simulink model "pcc_dynamic_model_actuation_dynamics"  (R2021a)
settings: Solver=VariableStepAuto  StartTime=0.0  StopTime=30  MaxStep=0.005  RelTol=1e-3
libraries: simulink x3, simulink_extras x3, pid_lib x1
settings Model: PauseTimes=0  Creator=maximilianstoelzle  LastModifiedBy=mstolzle

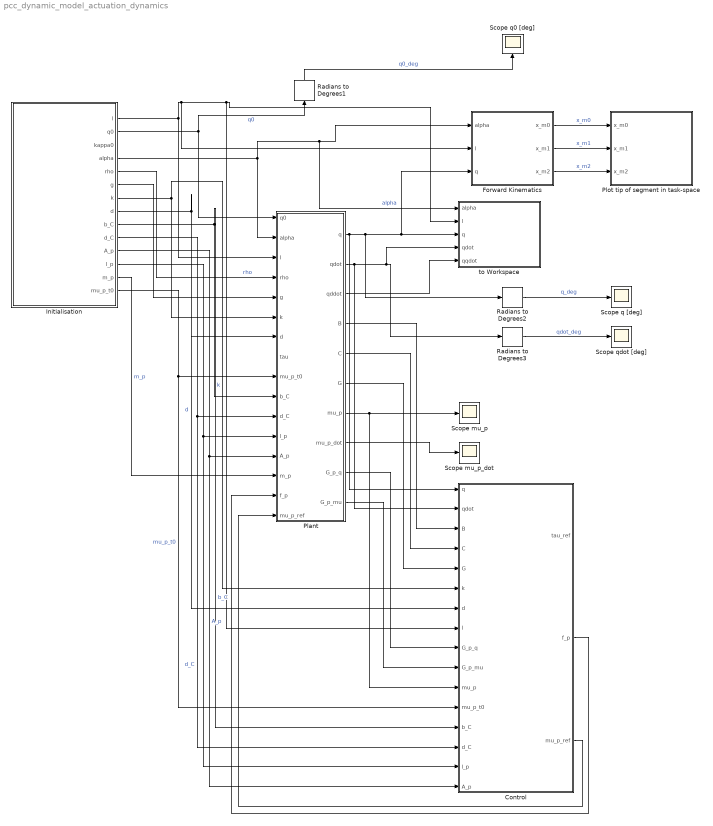
== system pcc_dynamic_model_actuation_dynamics ==
  Control : Subsystem
  Forward Kinematics : MATLAB Function  TreatAsAtomicUnit=on
  Initialisation : Subsystem
  Plant : Subsystem
  Plot tip of segment in task-space : Subsystem
  Radians to Degrees1 : simulink_extras/Transformations/Radians to Degrees
  Radians to Degrees2 : simulink_extras/Transformations/Radians to Degrees
  Radians to Degrees3 : simulink_extras/Transformations/Radians to Degrees
  Scope mu_p : Scope
  Scope mu_p_dot : Scope
  Scope q [deg] : Scope
  Scope q0 [deg] : Scope
  Scope qdot [deg] : Scope
  to Workspace : Subsystem
  wires:
  Initialisation/13(m_p) -> Plant/14(m_p)  "m_p"
  Plant/5(C) -> Control/4(C)
  Control/3(mu_p_ref) -> Plant/16(mu_p_ref)
  Initialisation/14(mu_p_t0) -> Plant/9(mu_p_t0), Control/12(mu_p_t0)  "mu_p_t0"
  Plant/10(G_p_mu) -> Control/10(G_p_mu)
  Initialisation/7(k) -> Plant/6(k), Control/6(k)  "k"
  Plant/8(mu_p_dot) -> Scope mu_p_dot/1
  Plant/9(G_p_q) -> Control/9(G_p_q)
  Control/2(f_p) -> Plant/15(f_p)
  Radians to Degrees1/1 -> Scope q0 [deg]/1  "q0_deg"
  Plant/6(G) -> Control/5(G)
  Plant/4(B) -> Control/3(B)
  Initialisation/6(g) -> Plant/5(g)
  Initialisation/5(rho) -> Plant/4(rho)  "rho"
  Plant/3(qddot) -> to Workspace/5(qqdot)
  Radians to Degrees3/1 -> Scope qdot [deg]/1  "qdot_deg"
  Forward Kinematics/3(x_m2) -> Plot tip of segment in task-space/3(x_m2)  "x_m2"
  Forward Kinematics/2(x_m1) -> Plot tip of segment in task-space/2(x_m1)  "x_m1"
  Forward Kinematics/1(x_m0) -> Plot tip of segment in task-space/1(x_m0)  "x_m0"
  Radians to Degrees2/1 -> Scope q [deg]/1  "q_deg"
  Plant/7(mu_p) -> Scope mu_p/1, Control/11(mu_p)
  Initialisation/12(l_p) -> Plant/12(l_p), Control/15(l_p)
  Initialisation/9(b_C) -> Plant/10(b_C), Control/13(b_C)  "b_C"
  Initialisation/10(d_C) -> Control/14(d_C), Plant/11(d_C)  "d_C"
  Initialisation/11(A_p) -> Control/16(A_p), Plant/13(A_p)  "A_p"
  Initialisation/2(q0) -> Plant/1(q0), Radians to Degrees1/1  "q0"
  Plant/1(q) -> Forward Kinematics/3(q), to Workspace/3(q), Radians to Degrees2/1, Control/1(q)
  Plant/2(qdot) -> to Workspace/4(qdot), Radians to Degrees3/1, Control/2(qdot)
  Initialisation/8(d) -> Control/7(d), Plant/7(d)  "d"
  Initialisation/4(alpha) -> Plant/2(alpha), to Workspace/1(alpha), Forward Kinematics/1(alpha)  "alpha"
  Initialisation/1(l) -> Plant/3(l), to Workspace/2(l), Control/8(l), Forward Kinematics/2(l)

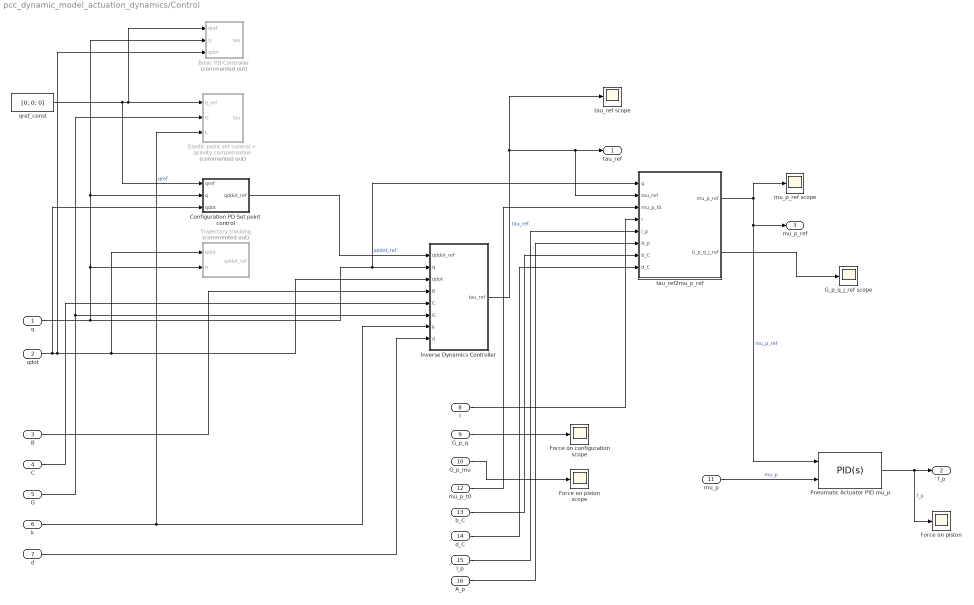
== system pcc_dynamic_model_actuation_dynamics/Control ==
  q : Inport
  qdot : Inport  Port=2
  B : Inport  Port=3
  C : Inport  Port=4
  G : Inport  Port=5
  k : Inport  Port=6
  d : Inport  Port=7
  l : Inport  Port=8
  G_p_q : Inport  Port=9
  G_p_mu : Inport  Port=10
  mu_p : Inport  Port=11
  mu_p_t0 : Inport  Port=12
  b_C : Inport  Port=13
  d_C : Inport  Port=14
  l_p : Inport  Port=15
  A_p : Inport  Port=16
  Basic PD Controller : Subsystem  Commented=on
  Configuration PD Set point control : Subsystem
  Elastic point set control + gravity compensation : MATLAB Function  Commented=on  TreatAsAtomicUnit=on
  Force on configuration scope : Scope
  Force on piston : Scope
  Force on piston scope : Scope
  G_p_q_j_ref scope : Scope
  Inverse Dynamics Controller : MATLAB Function  TreatAsAtomicUnit=on
  Pneumatic Actuator PID mu_p : pid_lib/PID Controller (2DOF)  Controller=PID  Form=Parallel  TimeDomain=Continuous-time  UseExternalTs=off  SampleTime=-1  IntegratorMethod=Forward Euler  FilterMethod=Forward Euler  ControllerParametersSource=internal  P=-3000  I=-500  D=-100  UseFilter=on  N=100  b=1  c=1  TunerSelectOption=Frequency Response Based  InitialConditionSource=internal  InitialConditionForIntegrator=0  InitialConditionForFilter=0  DifferentiatorICPrevScaledInput=0  ExternalReset=none  TrackingMode=off  Kt=1  LimitOutput=off  SatLimitsSource=internal  UpperSaturationLimit=inf  LowerSaturationLimit=-inf  LinearizeAsGain=on  AntiWindupMode=none  Kb=1  POutMin=[]  POutMax=[]  IOutMin=[]  IOutMax=[]  DOutMin=[]  DOutMax=[]  NOutMin=[]  NOutMax=[]  bOutMin=[]  bOutMax=[]  cOutMin=[]  cOutMax=[]  SumOutMin=[]  SumOutMax=[]  SaturationOutMin=[]  SaturationOutMax=[]  PParamMin=[]  PParamMax=[]  IParamMin=[]  IParamMax=[]  DParamMin=[]  DParamMax=[]  NParamMin=[]  NParamMax=[]  bParamMin=[]  bParamMax=[]  cParamMin=[]  cParamMax=[]  KbParamMin=[]  KbParamMax=[]  KtParamMin=[]  KtParamMax=[]  KbOutMin=[]  KbOutMax=[]  KtOutMin=[]  KtOutMax=[]  IntegratorOutMin=[]  IntegratorOutMax=[]  FilterOutMin=[]  FilterOutMax=[]  SumI1OutMin=[]  SumI1OutMax=[]  SumI2OutMin=[]  SumI2OutMax=[]  SumI3OutMin=[]  SumI3OutMax=[]  SumI4OutMin=[]  SumI4OutMax=[]  SumDOutMin=[]  SumDOutMax=[]  Sum1OutMin=[]  Sum1OutMax=[]  Sum2OutMin=[]  Sum2OutMax=[]  Sum3OutMin=[]  Sum3OutMax=[]  DifferentiatorOutMin=[]  DifferentiatorOutMax=[]  FilterDiffOutCoefMin=[]  FilterDiffOutCoefMax=[]  ReciprocalOutMin=[]  ReciprocalOutMax=[]  SumDenOutMin=[]  SumDenOutMax=[]  SumNumOutMin=[]  SumNumOutMax=[]  DivideOutMin=[]  DivideOutMax=[]  UdiffTsProdOutMin=[]  UdiffTsProdOutMax=[]  NTsProdOutMin=[]  NTsProdOutMax=[]  UintegralTsProdOutMin=[]  UintegralTsProdOutMax=[]  UngainTsProdOutMin=[]  UngainTsProdOutMax=[]  IntegratorContinuousStateAttributes=''  IntegratorStateMustResolveToSignalObject=off  IntegratorRTWStateStorageClass=Auto  FilterContinuousStateAttributes=''  FilterStateMustResolveToSignalObject=off  FilterRTWStateStorageClass=Auto  ParallelPVariant=InternalParameters  IdealPVariant=Disabled  IVariant=InternalParameters  DVariant=InternalParameters  bVariant=InternalParameters  cVariant=InternalParameters  IntegratorVariant=Continuous  SatVariant=Disabled  AWVariant=Passthrough  PCopyVariant=Disabled  TRVariant=Disabled  FdbkBlocksVariant=Forward  IdealPFdbkVariant=Disabled  SatFdbkVariant=Disabled  DerivativeFilterVariant=ContFilter  NVariant=InternalParameters  NCopyVariant=Disabled  FilterICVariant=InternalICsFilter  IntegratorICVariant=InternalICs  ExternalResetVariant=Disabled  TRSumVariant=Passthrough  SumFdbkVariant=Disabled  SumVariant=Sum_PID  TsampFilterVariant=InternalTs  TsampNgainVariant=Passthrough  TsampIntegralVariant=Passthrough  ExternalSaturationOutDataTypeStr=Inherit: Same as second input
      settings: SourceProductBaseCode=SL
  Trajectory tracking : Subsystem  Commented=on
  mu_p_ref scope : Scope
  qref_const : Constant  Value=[0; 0; 0]
  tau_ref scope : Scope
  tau_ref2mu_p_ref : MATLAB Function  TreatAsAtomicUnit=on
  tau_ref : Outport
  f_p : Outport  Port=2
  mu_p_ref : Outport  Port=3
  wires:
  q/1 -> Trajectory tracking/2(q), Configuration PD Set point control/2(q), Basic PD Controller/2(q), tau_ref2mu_p_ref/1(q), Inverse Dynamics Controller/2(q)
  qdot/1 -> Trajectory tracking/1(qdot), Inverse Dynamics Controller/3(qdot), Basic PD Controller/3(qdot), Configuration PD Set point control/3(qdot)
  B/1 -> Inverse Dynamics Controller/4(B)
  C/1 -> Inverse Dynamics Controller/5(C)
  G/1 -> Elastic point set control + gravity compensation/2(G), Inverse Dynamics Controller/6(G)
  k/1 -> Elastic point set control + gravity compensation/3(k), Inverse Dynamics Controller/7(k)
  d/1 -> Inverse Dynamics Controller/8(d)
  qref_const/1 -> Basic PD Controller/1(qref), Elastic point set control + gravity compensation/1(q_ref), Configuration PD Set point control/1(qref)  "qref"
  Configuration PD Set point control/1(qddot_ref) -> Inverse Dynamics Controller/1(qddot_ref)  "qddot_ref"
  Inverse Dynamics Controller/1(tau_ref) -> tau_ref2mu_p_ref/2(tau_ref), tau_ref/1, tau_ref scope/1  "tau_ref"
  Pneumatic Actuator PID mu_p/1 -> Force on piston/1, f_p/1  "f_p"
  mu_p/1 -> Pneumatic Actuator PID mu_p/2  "mu_p"
  tau_ref2mu_p_ref/1(mu_p_ref) -> Pneumatic Actuator PID mu_p/1, mu_p_ref/1, mu_p_ref scope/1  "mu_p_ref"
  mu_p_t0/1 -> tau_ref2mu_p_ref/3(mu_p_t0)
  b_C/1 -> tau_ref2mu_p_ref/7(b_C)
  d_C/1 -> tau_ref2mu_p_ref/8(d_C)
  l_p/1 -> tau_ref2mu_p_ref/5(l_p)
  A_p/1 -> tau_ref2mu_p_ref/6(A_p)
  l/1 -> tau_ref2mu_p_ref/4(l)
  tau_ref2mu_p_ref/2(G_p_q_j_ref) -> G_p_q_j_ref scope/1
  G_p_q/1 -> Force on configuration scope/1
  G_p_mu/1 -> Force on piston scope/1

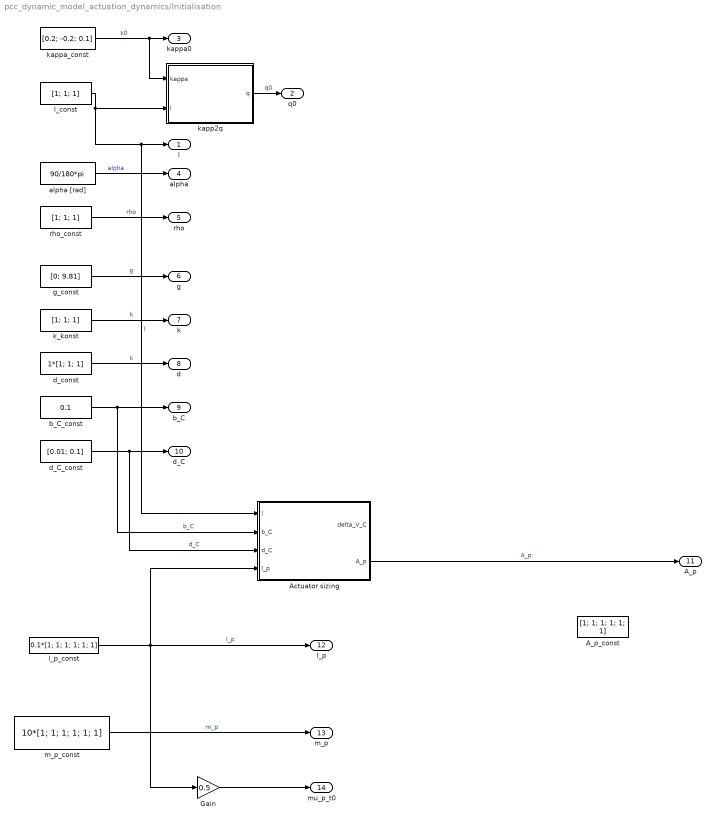
== system pcc_dynamic_model_actuation_dynamics/Initialisation ==
  A_p_const : Constant  Value=[1; 1; 1; 1; 1; 1]
  Actuator sizing : MATLAB Function  TreatAsAtomicUnit=on
  Gain : Gain  Gain=0.5
  alpha [rad] : Constant  Value=90/180*pi
  b_C_const : Constant  Value=0.1
  d_C_const : Constant  Value=[0.01; 0.1]
  d_const : Constant  Value=1*[1; 1; 1]
  g_const : Constant  Value=[0; 9.81]
  k_konst : Constant  Value=[1; 1; 1]
  kapp2q : MATLAB Function  TreatAsAtomicUnit=on
  kappa_const : Constant  Value=[0.2; -0.2; 0.1]
  l_const : Constant  Value=[1; 1; 1]
  l_p_const : Constant  Value=0.1*[1; 1; 1; 1; 1; 1]
  m_p_const : Constant  Value=10*[1; 1; 1; 1; 1; 1]
  rho_const : Constant  Value=[1; 1; 1]
  l : Outport
  q0 : Outport  Port=2
  kappa0 : Outport  Port=3
  alpha : Outport  Port=4
  rho : Outport  Port=5
  g : Outport  Port=6
  k : Outport  Port=7
  d : Outport  Port=8
  b_C : Outport  Port=9
  d_C : Outport  Port=10
  A_p : Outport  Port=11
  l_p : Outport  Port=12
  m_p : Outport  Port=13
  mu_p_t0 : Outport  Port=14
  wires:
  kappa_const/1 -> kapp2q/1(kappa), kappa0/1  "k0"
  l_const/1 -> kapp2q/2(l), Actuator sizing/1(l), l/1  "l"
  alpha [rad]/1 -> alpha/1  "alpha"
  kapp2q/1(q) -> q0/1  "q0"
  rho_const/1 -> rho/1  "rho"
  g_const/1 -> g/1  "g"
  k_konst/1 -> k/1  "k"
  d_const/1 -> d/1  "k"
  d_C_const/1 -> Actuator sizing/3(d_C), d_C/1  "d_C"
  m_p_const/1 -> m_p/1  "m_p"
  b_C_const/1 -> Actuator sizing/2(b_C), b_C/1  "b_C"
  l_p_const/1 -> Gain/1, Actuator sizing/4(l_p), l_p/1  "l_p"
  Actuator sizing/2(A_p) -> A_p/1  "A_p"
  Gain/1 -> mu_p_t0/1

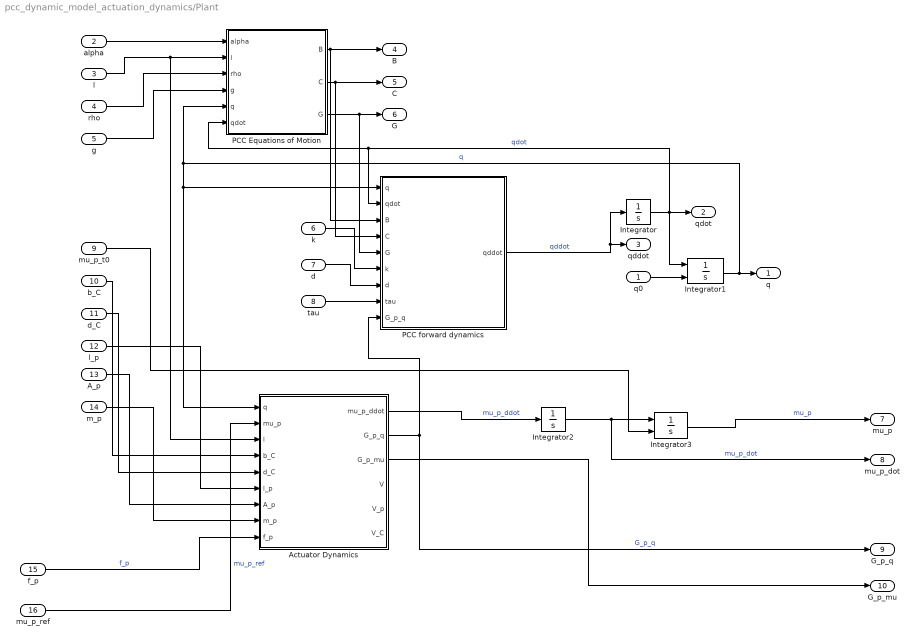
== system pcc_dynamic_model_actuation_dynamics/Plant ==
  q0 : Inport
  alpha : Inport  Port=2
  l : Inport  Port=3
  rho : Inport  Port=4
  g : Inport  Port=5
  k : Inport  Port=6
  d : Inport  Port=7
  tau : Inport  Port=8
  mu_p_t0 : Inport  Port=9
  b_C : Inport  Port=10
  d_C : Inport  Port=11
  l_p : Inport  Port=12
  A_p : Inport  Port=13
  m_p : Inport  Port=14
  f_p : Inport  Port=15
  mu_p_ref : Inport  Port=16
  Actuator Dynamics : MATLAB Function  TreatAsAtomicUnit=on
  Integrator : Integrator  InitialCondition=[0; 0; 0]
  Integrator1 : Integrator  InitialConditionSource=external
  Integrator2 : Integrator  InitialCondition=[0; 0; 0; 0; 0; 0]
  Integrator3 : Integrator  InitialConditionSource=external  LimitOutput=on  UpperSaturationLimit=0.1*[1; 1; 1; 1; 1; 1]  LowerSaturationLimit=[0; 0; 0; 0; 0; 0]
  PCC Equations of Motion : MATLAB Function  TreatAsAtomicUnit=on
  PCC forward dynamics : MATLAB Function  TreatAsAtomicUnit=on
  q : Outport
  qdot : Outport  Port=2
  qddot : Outport  Port=3
  B : Outport  Port=4
  C : Outport  Port=5
  G : Outport  Port=6
  mu_p : Outport  Port=7
  mu_p_dot : Outport  Port=8
  G_p_q : Outport  Port=9
  G_p_mu : Outport  Port=10
  wires:
  g/1 -> PCC Equations of Motion/4(g)
  alpha/1 -> PCC Equations of Motion/1(alpha)
  q0/1 -> Integrator1/2
  k/1 -> PCC forward dynamics/6(k)
  l/1 -> Actuator Dynamics/3(l), PCC Equations of Motion/2(l)
  PCC Equations of Motion/3(G) -> PCC forward dynamics/5(G), G/1
  PCC Equations of Motion/1(B) -> PCC forward dynamics/3(B), B/1
  Integrator1/1 -> PCC Equations of Motion/5(q), Actuator Dynamics/1(q), PCC forward dynamics/1(q), q/1  "q"
  PCC forward dynamics/1(qddot) -> Integrator/1, qddot/1  "qddot"
  rho/1 -> PCC Equations of Motion/3(rho)
  d/1 -> PCC forward dynamics/7(d)
  Integrator/1 -> PCC forward dynamics/2(qdot), PCC Equations of Motion/6(qdot), Integrator1/1, qdot/1  "qdot"
  PCC Equations of Motion/2(C) -> PCC forward dynamics/4(C), C/1
  A_p/1 -> Actuator Dynamics/7(A_p)
  m_p/1 -> Actuator Dynamics/8(m_p)
  Actuator Dynamics/1(mu_p_ddot) -> Integrator2/1  "mu_p_ddot"
  d_C/1 -> Actuator Dynamics/5(d_C)
  Integrator2/1 -> Integrator3/1, mu_p_dot/1  "mu_p_dot"
  b_C/1 -> Actuator Dynamics/4(b_C)
  l_p/1 -> Actuator Dynamics/6(l_p)
  Integrator3/1 -> mu_p/1  "mu_p"
  Actuator Dynamics/2(G_p_q) -> G_p_q/1, PCC forward dynamics/9(G_p_q)  "G_p_q"
  tau/1 -> PCC forward dynamics/8(tau)
  Actuator Dynamics/3(G_p_mu) -> G_p_mu/1
  f_p/1 -> Actuator Dynamics/9(f_p)  "f_p"
  mu_p_t0/1 -> Integrator3/2
  mu_p_ref/1 -> Actuator Dynamics/2(mu_p)  "mu_p_ref"

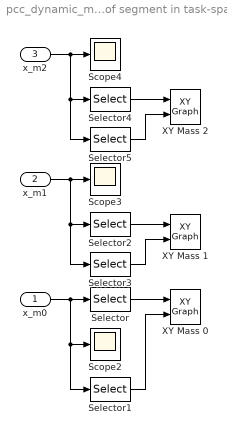
== system pcc_dynamic_model_actuation_dynamics/Plot tip of segment in task-space ==
  x_m0 : Inport
  x_m1 : Inport  Port=2
  x_m2 : Inport  Port=3
  Scope2 : Scope
  Scope3 : Scope
  Scope4 : Scope
  Selector : Selector  InputPortWidth=2  IndexOptions=Index vector (dialog)  Indices=[1]  OutputSizes=1
  Selector1 : Selector  InputPortWidth=2  IndexOptions=Index vector (dialog)  Indices=[2]  OutputSizes=1
  Selector2 : Selector  InputPortWidth=2  IndexOptions=Index vector (dialog)  Indices=[1]  OutputSizes=1
  Selector3 : Selector  InputPortWidth=2  IndexOptions=Index vector (dialog)  Indices=[2]  OutputSizes=1
  Selector4 : Selector  InputPortWidth=2  IndexOptions=Index vector (dialog)  Indices=[1]  OutputSizes=1
  Selector5 : Selector  InputPortWidth=2  IndexOptions=Index vector (dialog)  Indices=[2]  OutputSizes=1
  XY Mass 0 : simulink/Sinks/XY Graph  xmin=-10  xmax=10  ymin=-10  ymax=10  st=-1
  XY Mass 1 : simulink/Sinks/XY Graph  xmin=-10  xmax=10  ymin=-10  ymax=10  st=-1
  XY Mass 2 : simulink/Sinks/XY Graph  xmin=-10  xmax=10  ymin=-10  ymax=10  st=-1
  wires:
  x_m2/1 -> Selector5/1, Selector4/1, Scope4/1
  Selector/1 -> XY Mass 0/1
  x_m1/1 -> Selector3/1, Selector2/1, Scope3/1
  Selector5/1 -> XY Mass 2/2
  Selector3/1 -> XY Mass 1/2
  Selector1/1 -> XY Mass 0/2
  x_m0/1 -> Scope2/1, Selector1/1, Selector/1
  Selector4/1 -> XY Mass 2/1
  Selector2/1 -> XY Mass 1/1

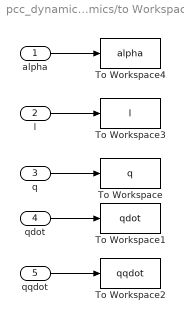
== system pcc_dynamic_model_actuation_dynamics/to Workspace ==
  alpha : Inport
  l : Inport  Port=2
  q : Inport  Port=3
  qdot : Inport  Port=4
  qqdot : Inport  Port=5
  To Workspace : ToWorkspace  VariableName=q  SaveFormat=Timeseries  SampleTime=-1
  To Workspace1 : ToWorkspace  VariableName=qdot  SaveFormat=Timeseries  SampleTime=-1
  To Workspace2 : ToWorkspace  VariableName=qqdot  SaveFormat=Timeseries  SampleTime=-1
  To Workspace3 : ToWorkspace  VariableName=l  SaveFormat=Timeseries  SampleTime=-1
  To Workspace4 : ToWorkspace  VariableName=alpha  SaveFormat=Timeseries  SampleTime=-1
  wires:
  alpha/1 -> To Workspace4/1
  qdot/1 -> To Workspace1/1
  l/1 -> To Workspace3/1
  qqdot/1 -> To Workspace2/1
  q/1 -> To Workspace/1

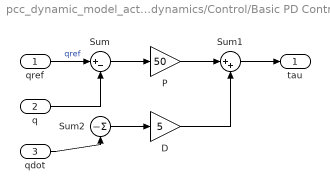
== system pcc_dynamic_model_actuation_dynamics/Control/Basic PD Controller ==
  qref : Inport
  q : Inport  Port=2
  qdot : Inport  Port=3
  D : Gain  Gain=5
  P : Gain  Gain=50
  Sum : Sum  Inputs=|+-
  Sum1 : Sum  Inputs=|++
  Sum2 : Sum  Inputs=||-
  tau : Outport
  wires:
  qdot/1 -> Sum2/1
  Sum1/1 -> tau/1
  D/1 -> Sum1/2
  q/1 -> Sum/2
  qref/1 -> Sum/1  "qref"
  Sum/1 -> P/1
  P/1 -> Sum1/1
  Sum2/1 -> D/1

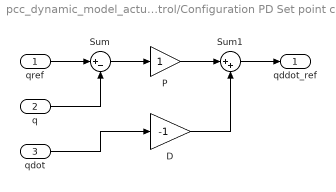
== system pcc_dynamic_model_actuation_dynamics/Control/Configuration PD Set point control ==
  qref : Inport
  q : Inport  Port=2
  qdot : Inport  Port=3
  D : Gain  Gain=-1
  P : Gain
  Sum : Sum  Inputs=|+-
  Sum1 : Sum  Inputs=|++
  qddot_ref : Outport
  wires:
  Sum1/1 -> qddot_ref/1
  D/1 -> Sum1/2
  q/1 -> Sum/2
  qref/1 -> Sum/1
  Sum/1 -> P/1
  P/1 -> Sum1/1
  qdot/1 -> D/1

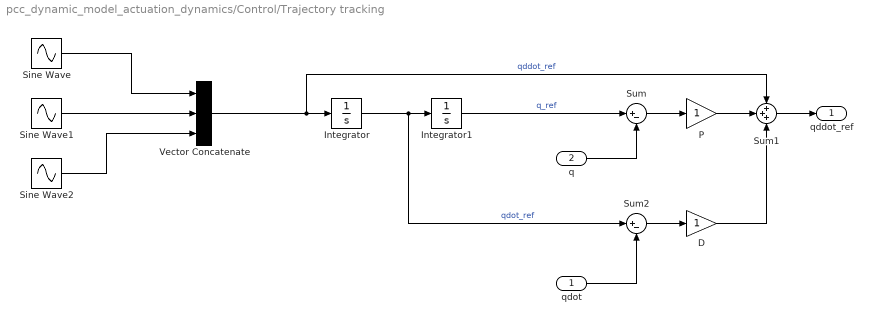
== system pcc_dynamic_model_actuation_dynamics/Control/Trajectory tracking ==
  qdot : Inport
  q : Inport  Port=2
  D : Gain
  Integrator : Integrator  InitialCondition=[-0.25, -0.5, -1]
  Integrator1 : Integrator
  P : Gain
  Sine Wave : Sin  Amplitude=0.25  Samples=100  SampleTime=0
  Sine Wave1 : Sin  Amplitude=0.5  SampleTime=0
  Sine Wave2 : Sin  SampleTime=0
  Sum : Sum  Inputs=|+-
  Sum1 : Sum  Inputs=+++
  Sum2 : Sum  Inputs=|+-
  Vector Concatenate : Concatenate  NumInputs=3
  qddot_ref : Outport
  wires:
  Sum1/1 -> qddot_ref/1
  q/1 -> Sum/2
  Sum/1 -> P/1
  Vector Concatenate/1 -> Sum1/1, Integrator/1  "qddot_ref"
  Integrator/1 -> Sum2/1, Integrator1/1  "qdot_ref"
  Integrator1/1 -> Sum/1  "q_ref"
  qdot/1 -> Sum2/2
  Sum2/1 -> D/1
  D/1 -> Sum1/3
  P/1 -> Sum1/2
  Sine Wave/1 -> Vector Concatenate/1
  Sine Wave1/1 -> Vector Concatenate/2
  Sine Wave2/1 -> Vector Concatenate/3

== matlab function pcc_dynamic_model_actuation_dynamics/Initialisation/Actuator sizing ==
  data: l input; delta_V_C output; b_C input; d_C input; l_p input; A_p output
function [delta_V_C, A_p]= piston_sizing(l, b_C, d_C, l_p)
    q_min = -90/180*pi*ones(length(l), 1);
    q_max = 90/180*pi*ones(length(l), 1);
    delta_V_C = abs(V_C_fun(q_max, l, b_C, d_C) - V_C_fun(q_min, l, b_C, d_C));
    A_p = 1*delta_V_C ./ l_p;
end

== matlab function pcc_dynamic_model_actuation_dynamics/Control/tau_ref2mu_p_ref ==
  data: q input; tau_ref input; mu_p_ref output; mu_p_t0 input; l input; l_p input; A_p input; b_C input; d_C input; G_p_q_j_ref output
function [mu_p_ref, G_p_q_j_ref]= tau_ref2mu_p_ref(q, tau_ref, mu_p_t0, l, l_p, A_p, b_C, d_C)
    mu_p_ref = mu_p_ref_fun(q, tau_ref, mu_p_t0, l, l_p, A_p, b_C, d_C);
    G_p_q_j_ref = G_p_q_j_ref_fun(tau_ref, mu_p_t0, l, l_p, A_p, b_C, d_C);
end

== matlab function pcc_dynamic_model_actuation_dynamics/Forward Kinematics ==
  data: alpha input; x_m0 output; l input; q input; x_m1 output; x_m2 output
function [x_m0, x_m1, x_m2] = forward_kinematics(alpha, l, q)
    x_m0 = q2x0_fun(l(1), q, alpha, l);
    x_m1 = q2x1_fun(l(2), q, alpha, l);
    x_m2 = q2x2_fun(l(3), q, alpha, l);
end

== matlab function pcc_dynamic_model_actuation_dynamics/Plant/PCC forward dynamics ==
  data: q input; qdot input; B input; qddot output; C input; G input; k input; d input; tau input; G_p_q input
function qddot  = pcc_forward_dynamics(q, qdot, B, C, G, k, d, tau, G_p_q)
    pinv_tol = 0.0001;
    qddot = pinv(B, pinv_tol)*(-(C*qdot)-G-(k.*q)-(d.*qdot)-G_p_q+tau);
end

== matlab function pcc_dynamic_model_actuation_dynamics/Initialisation/kapp2q ==
  data: kappa input; q output; l input
function q = kappa2q(kappa, l)
    q = [kappa(1) * l(1);
         kappa(2) * l(2);
         kappa(3) * l(3)];
end

== matlab function pcc_dynamic_model_actuation_dynamics/Plant/PCC Equations of Motion ==
  data: alpha input; l input; rho input; B output; g input; q input; qdot input; C output; G output
function [B, C, G]  = pcc_eom(alpha, l, rho, g, q, qdot)
    n_b = length(l);
  
    % introduce tolerance for numerical stability
    tol = 0.005;
    for i=1:n_b
        if 0 <= q(i) && q(i) < tol
            q(i) = tol;
        elseif q(i) < 0 && -tol < q(i)
            q(i) = -tol;
        end
    end
    
%     Bi = zeros(n_b, n_b, n_b);
%     for i=1:n_b
%         s_dash = tol;
%         ds = l(i) / 50;
%         while s_dash < l(1)
%             if i == 1
%                 dBi_sdash = B0_ds_fun(s_dash, q, alpha, l, rho);
%             elseif i == 2
%                 dBi_sdash = B1_ds_fun(s_dash, q, alpha, l, rho);
%             else
%                 dBi_sdash = B2_ds_fun(s_dash, q, alpha, l, rho);
%             end
%             Bi(i, :, :) = squeeze(Bi(i, :, :)) + dBi_sdash*ds;
%             s_dash = s_dash + ds;
%         end
%     end
%     B = squeeze(sum(Bi, 1));
    B = B_fun(q, alpha, l, rho);
    
    C = C_fun(q, qdot, alpha, l, rho);
%     C = zeros(n_b, n_b);
%     C(1,1) = C11_fun(q, qdot, alpha, l, rho);
%     C(1,2) = C12_fun(q, qdot, alpha, l, rho);
%     C(1,3) = C13_fun(q, qdot, alpha, l, rho);
%     C(2,1) = C21_fun(q, qdot, alpha, l, rho);
%     C(2,2) = C22_fun(q, qdot, alpha, l, rho);
%     C(2,3) = C23_fun(q, qdot, alpha, l, rho);
%     C(3,1) = C31_fun(q, qdot, alpha, l, rho);
%     C(3,2) = C32_fun(q, qdot, alpha, l, rho);
%     C(3,3) = C33_fun(q, qdot, alpha, l, rho);
    
    G = G_fun(q, alpha, l, rho, g);
end

== matlab function pcc_dynamic_model_actuation_dynamics/Control/Inverse Dynamics Controller ==
  data: qddot_ref input; q input; tau_ref output; qdot input; B input; C input; G input; k input; d input
function tau_ref = fcn(qddot_ref, q, qdot, B, C, G, k, d)
    tau_ref = B*qddot_ref + C*qdot + G + k.*q + d.*qdot;
end

== matlab function pcc_dynamic_model_actuation_dynamics/Control/Elastic point set control + gravity compensation ==
  data: q_ref input; tau output; G input; k input
function tau = fcn(q_ref, G, k)
    tau = k.*q_ref + G;
end

== matlab function pcc_dynamic_model_actuation_dynamics/Plant/Actuator Dynamics ==
  data: mu_p_ddot output; q input; mu_p input; l input; b_C input; d_C input; l_p input; A_p input; G_p_q output; G_p_mu output; m_p input; f_p input; V output; V_p output; V_C output
function [mu_p_ddot, G_p_q, G_p_mu, V, V_p, V_C]  = actuator_dynamics(q, mu_p, l, b_C, d_C, l_p, A_p, m_p, f_p)
    % introduce tolerance for numerical stability
%     tol = 0.005;
%     for j=1:length(mu_p)
%         if mu_p(j) < tol
%             mu_p(j) = tol;
%         end
%     end
    
    % volume of fluid
    V = V_fun(q, mu_p, l, A_p, b_C, d_C);
    V_p = V_p_fun(mu_p, A_p);
    V_C = V_C_fun(q, l, b_C, d_C);

    % potential forces by fluid
    G_p_q = G_p_q_fun(q, mu_p, l, l_p, A_p, b_C, d_C);
    G_p_mu = G_p_mu_fun(q, mu_p, l, l_p, A_p, b_C, d_C);
    
    
    M_p = diag(m_p);
    
    pinv_tol = 0.0001;
    mu_p_ddot = pinv(M_p, pinv_tol)*(-G_p_mu-f_p);
end
